simulink model "qnd_chirp"  (R2021a)
settings: Solver=VariableStepAuto  StartTime=0.0  StopTime=Tsweep  RelTol=1e-3
PreLoadFcn:
  | preload_fcn
values from neighbouring files (symbols this model uses):
  BW = 10e3    (= 10000)    [preload_fcn.m]
  Fs = OSR*BW    (= 25600)    [preload_fcn.m]
  H = tf([1 0 (2*pi*1e3)^2],[1 2*pi*1e3 (2*pi*1e3)^2])    [preload_fcn.m]
libraries: dsparch4 x1, dspsrcs4 x1
settings Model: NumberOfSteps=1000  Creator=kschutz  LastModifiedBy=kschutz

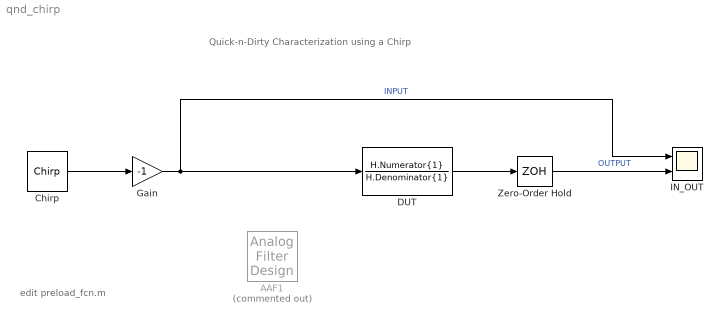
== system qnd_chirp ==
  note: Quick-n-Dirty Characterization using a Chirp
  note: edit preload_fcn.m
  AAF1 : dsparch4/Analog Filter Design  Commented=on  method=Elliptic  filttype=Lowpass  N=8  Wlo=2*pi*BW  Whi=80  Rp=.5  Rs=80
  Chirp : dspsrcs4/Chirp  sweep=Linear  mode=Unidirectional  f0=0  f1=BW  t1=Tsweep  Tsweep=Tsweep  phase=pi/2  Ts=1/(Fs)  spf=1  datatype=Double  OutputFrames=off
      settings: AttributesFormatString=|
      | F_start =  %<f0>
      | F_stop = %<f1>
  DUT : TransferFcn  Numerator=H.Numerator{1}  Denominator=H.Denominator{1}
  Gain : Gain  Gain=-1
  IN_OUT : Scope  NumInputPorts=2
  Zero-Order Hold : ZeroOrderHold  SampleTime=1/(Fs)
  wires:
  Zero-Order Hold/1 -> IN_OUT/2  "OUTPUT"
  DUT/1 -> Zero-Order Hold/1
  Chirp/1 -> Gain/1
  Gain/1 -> DUT/1, IN_OUT/1  "INPUT"
